simulink model "circuitoA"  (R2021a)
settings: Solver=VariableStepAuto  StartTime=0.0  StopTime=10.0  RelTol=1e-3
model workspace (MAT data in the model file):
  Vi = 1
settings Model: Creator=phcs  LastModifiedBy=phcs

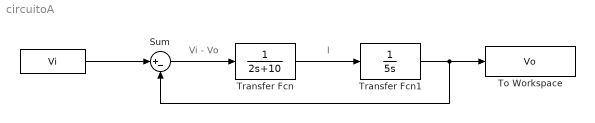
== system circuitoA ==
  note: I
  note: Vi - Vo
  " " : FromWorkspace  VariableName=Vi
  Sum : Sum  Inputs=|+-
  To Workspace : ToWorkspace  VariableName=Vo  SaveFormat=Timeseries  SampleTime=-1
  Transfer Fcn : TransferFcn  Denominator=[2 10]
  Transfer Fcn1 : TransferFcn  Denominator=[5 0]
  wires:
  " "/1 -> Sum/1
  Sum/1 -> Transfer Fcn/1
  Transfer Fcn/1 -> Transfer Fcn1/1
  Transfer Fcn1/1 -> Sum/2, To Workspace/1
